simulink model "single_track_ctrl_sim"  (R2018b)
settings: Solver=ode45  StartTime=0.0  StopTime=30  MaxStep=0.001  RelTol=1e-3
values from neighbouring files (symbols this model uses):
  A = [ 0,                     1,      vx,                           0 ... (first row only)    [single_ctrl_est_design.m]
  B = [0 c1/m 0 (a*c1)/J]'    [single_ctrl_est_design.m]
  vx = 7/3.6    (= 1.94444444444)    [single_ctrl_est_design.m]
libraries: simulink_extras x1, simulink x1
settings Model: Creator=jofr  LastModifiedBy=jossan
settings DataIOCC: LimitDataPoints=on  SaveFormat=Array  SignalLoggingSaveFormat=ModelDataLogs
settings OptimizationCC: BlockReduction=off  BooleanDataType=off  LifeSpan=inf
settings DebuggingCC: SaveWithParameterizedLinksMsg=none  UnderspecifiedInitializationDetection=Classic  MergeDetectMultiDrivingBlocksExec=none  SignalResolutionControl=TryResolveAllWithWarning  MultiTaskDSMMsg=warning  MultiTaskCondExecSysMsg=none  SFUnexpectedBacktrackingDiag=warning  SFNoUnconditionalDefaultTransitionDiag=warning  SFExecutionAtInitializationDiag=none
settings HardwareCC: ProdBitPerPointer=32  ProdBitPerSizeT=32  ProdBitPerPtrDiffT=32  ProdLargestAtomicFloat=None  ProdIntDivRoundTo=Undefined  ProdEndianess=Unspecified  ProdWordSize=32  ProdHWDeviceType=32-bit Generic  TargetUnknown=on
settings ModelReferenceCC: PropagateSignalLabelsOutOfModel=off
settings SFSimCC: SimUseLocalCustomCode=off
settings RTWCC: RTWUseLocalCustomCode=off
settings CodeAppCC: StateflowObjectComments=on
settings GRTTargetCC: TargetLangStandard=C89/C90 (ANSI)  GeneratePreprocessorConditionals=Disable all
settings ConfigComp: CovMetricSettings=dw  CovHtmlReporting=on  CovSaveCumulativeToWorkspaceVar=on  CovSaveSingleToWorkspaceVar=on  CovExternalEMLEnable=off

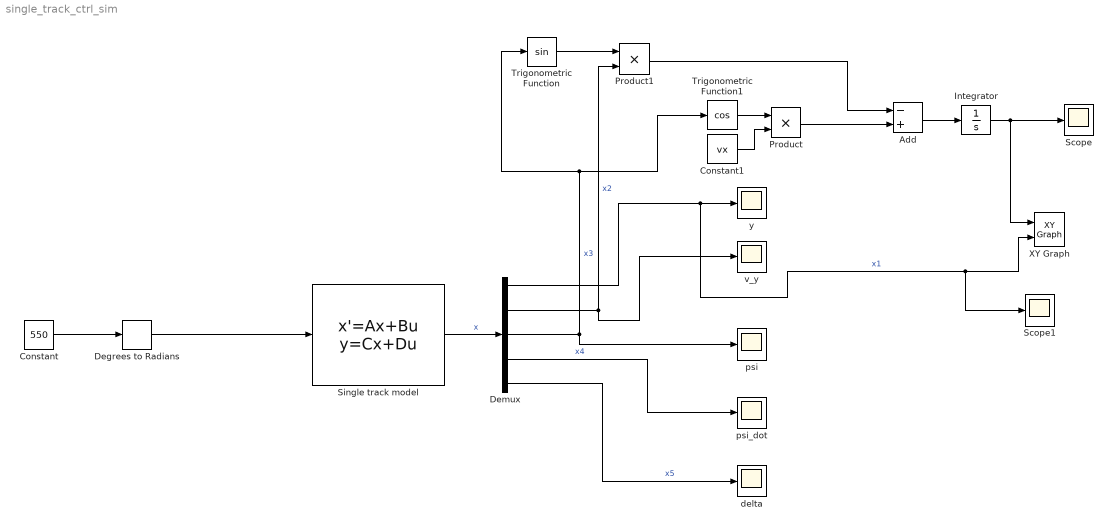
== system single_track_ctrl_sim ==
  Add : Sum  Inputs=-+
  Constant : Constant  Value=550
  Constant1 : Constant  Value=vx
  Degrees to Radians : simulink_extras/Transformations/Degrees to Radians
  Demux : Demux  Outputs=5
  Integrator : Integrator
  Product : Product
  Product1 : Product
  Scope : Scope
  Scope1 : Scope
  Single track model : StateSpace  A=A  B=B  C=eye(5)  D=zeros(5,1)  InitialCondition=0
  Trigonometric Function : Trigonometry
  Trigonometric Function1 : Trigonometry  Operator=cos
  XY Graph : simulink/Sinks/XY Graph  xmin=-20  xmax=20  ymin=-20  ymax=20  st=-1
  delta : Scope
  psi : Scope
  psi_dot : Scope
  v_y : Scope
  y : Scope
  wires:
  Single track model/1 -> Demux/1  "x"
  Demux/1 -> Scope1/1, XY Graph/2, y/1  "x1"
  Demux/2 -> v_y/1, Product1/2  "x2"
  Demux/3 -> psi/1, Trigonometric Function1/1, Trigonometric Function/1  "x3"
  Demux/4 -> psi_dot/1  "x4"
  Demux/5 -> delta/1  "x5"
  Constant/1 -> Degrees to Radians/1
  Degrees to Radians/1 -> Single track model/1
  Trigonometric Function1/1 -> Product/1
  Constant1/1 -> Product/2
  Trigonometric Function/1 -> Product1/1
  Product/1 -> Add/2
  Product1/1 -> Add/1
  Add/1 -> Integrator/1
  Integrator/1 -> XY Graph/1, Scope/1
